simulink model "Controlador_Cascada_RMS"  (R2020a)
settings: Solver=VariableStepAuto  StartTime=0.0  StopTime=10.0  MaxStep=0.0001  RelTol=1e-3
undefined symbols (not defined in the file): Amp, ba, bm, f, K_motor, K_motor_virtual, k_resorte, ksi, ksia, L, m_total, R, R_control
libraries: dspstat3 x1
settings Model: Creator=Adriana  LastModifiedBy=Noxi-PC

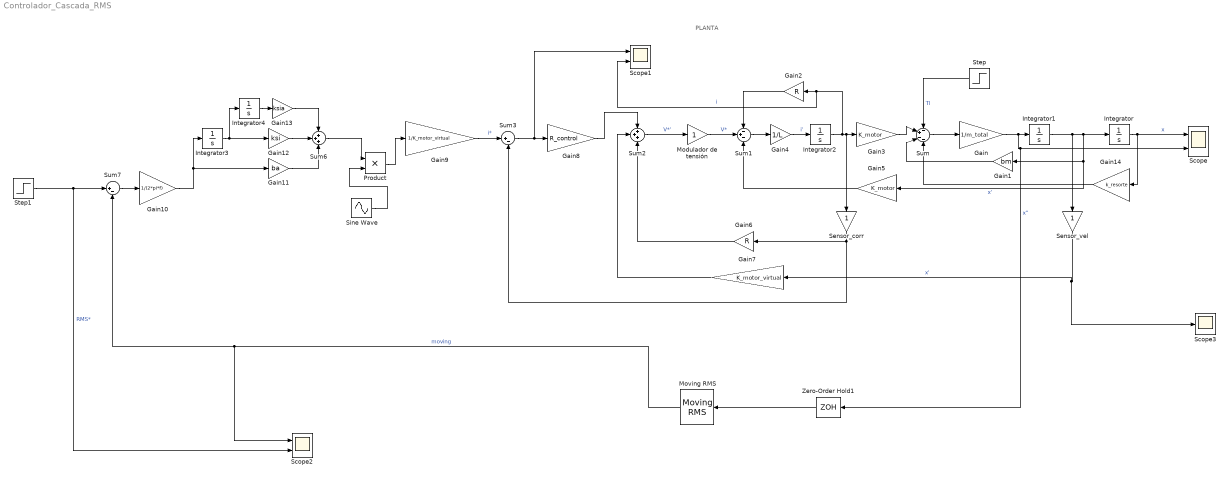
== system Controlador_Cascada_RMS ==
  note: PLANTA
  " Sensor_vel" : Gain
  Gain : Gain  Gain=1/m_total
  Gain1 : Gain  Gain=bm
  Gain10 : Gain  Gain=1/(2*pi*f)
  Gain11 : Gain  Gain=ba
  Gain12 : Gain  Gain=ksi
  Gain13 : Gain  Gain=ksia
  Gain14 : Gain  Gain=k_resorte
  Gain2 : Gain  Gain=R
  Gain3 : Gain  Gain=K_motor
  Gain4 : Gain  Gain=1/L
  Gain5 : Gain  Gain=K_motor
  Gain6 : Gain  Gain=R
  Gain7 : Gain  Gain=K_motor_virtual
  Gain8 : Gain  Gain=R_control
  Gain9 : Gain  Gain=1/K_motor_virtual
  Integrator{,1..4} (5 alike) : Integrator
  Modulador de tensión : Gain
  Moving RMS : dspstat3/Moving RMS  Method=Sliding window  ForgettingFactorPort=off  SpecifyWindowLength=on  WindowLength=Ventana  ForgettingFactor=0.99  SimulateUsing=Code generation
      settings: SourceProductBaseCode=DS
  Product : Product
  Scope : Scope  NumInputPorts=2
  Scope1 : Scope  NumInputPorts=2
  Scope2 : Scope  NumInputPorts=2
  Scope3 : Scope
  Sensor_corr : Gain
  Sine Wave : Sin  Frequency=2*pi*f  SampleTime=0
  Step : Step  Time=3  SampleTime=0
  Step1 : Step  After=Amp/sqrt(2)  SampleTime=0
  Sum : Sum  Inputs=-+--
  Sum1 : Sum  Inputs=-+-
  Sum2 : Sum  Inputs=+++
  Sum3 : Sum  Inputs=|+-
  Sum6 : Sum  Inputs=+++
  Sum7 : Sum  Inputs=|+-
  Zero-Order Hold1 : ZeroOrderHold  SampleTime=-1
  wires:
  Integrator1/1 -> " Sensor_vel"/1, Gain5/1, Gain1/1, Integrator/1  "x'"
  Integrator/1 -> Gain14/1, Scope/1  "x"
  Gain/1 -> Scope/2, Zero-Order Hold1/1, Integrator1/1  "x''"
  Sum/1 -> Gain/1
  Gain1/1 -> Sum/3
  Step/1 -> Sum/1  "Tl"
  Gain3/1 -> Sum/2
  Integrator2/1 -> Scope1/2, Gain2/1, Gain3/1, Sensor_corr/1  "i"
  Sum1/1 -> Gain4/1
  Gain4/1 -> Integrator2/1  "i'"
  Gain2/1 -> Sum1/1
  Gain5/1 -> Sum1/3
  Modulador de tensión/1 -> Sum1/2  "V*"
  Sum2/1 -> Modulador de tensión/1  "V*'"
  " Sensor_vel"/1 -> Scope3/1, Gain7/1  "x'"
  Sensor_corr/1 -> Sum3/2, Gain6/1
  Gain6/1 -> Sum2/3
  Gain7/1 -> Sum2/2
  Gain8/1 -> Sum2/1
  Sum3/1 -> Scope1/1, Gain8/1
  Gain9/1 -> Sum3/1  "i*"
  Integrator4/1 -> Gain13/1
  Integrator3/1 -> Integrator4/1, Gain12/1
  Gain12/1 -> Sum6/2
  Gain13/1 -> Sum6/1
  Sum7/1 -> Gain10/1
  Gain11/1 -> Sum6/3
  Gain14/1 -> Sum/4
  Moving RMS/1 -> Scope2/1, Sum7/2  "moving"
  Zero-Order Hold1/1 -> Moving RMS/1
  Step1/1 -> Scope2/2, Sum7/1  "RMS*"
  Gain10/1 -> Integrator3/1, Gain11/1
  Sum6/1 -> Product/1
  Product/1 -> Gain9/1
  Sine Wave/1 -> Product/2
